simulink model "bh_motor_test_speed_and_thrust_RPS"  (R2016a)
settings: Solver=ode23s  StartTime=0.0  StopTime=10  FixedStep=0.001  RelTol=1e-5
undefined symbols (not defined in the file): P_mot, P_mot_alone, P_one_prop, sigbuilder_block
libraries: bh_6dof_LIBRARY x6
settings Model: Creator=bhorton  LastModifiedBy=bhorton
settings DataIOCC: SaveOutput=off  SignalLogging=off  DSMLogging=off  VisualizeSimOutput=off  SaveTime=off
settings DebuggingCC: AlgebraicLoopMsg=error  AllowSymbolicDim=off
settings ModelReferenceCC: PropagateSignalLabelsOutOfModel=off
settings GRTTargetCC: GeneratePreprocessorConditionals=Use local settings

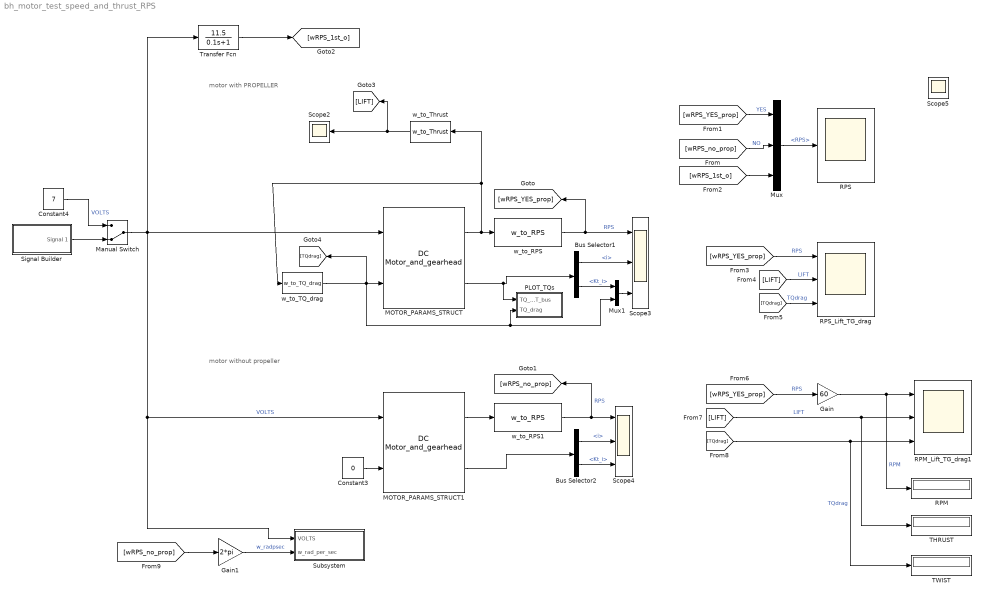
== system bh_motor_test_speed_and_thrust_RPS ==
  note: motor with PROPELLER
  note: motor without propeller
  Bus Selector1 : BusSelector  OutputSignals=Elec.i,TQ_mot.Kt_i
  Bus Selector2 : BusSelector  OutputSignals=Elec.i,TQ_mot.Kt_i
  Constant3 : Constant  Value=0
  Constant4 : Constant  Value=7
  Gain : Gain  Gain=60
  Gain1 : Gain  Gain=2*pi
  MOTOR_PARAMS_STRUCT : bh_6dof_LIBRARY/MODELS/DC Motor_and_gearhead  K=P_mot.Ka  B=P_mot.b  J=P_mot.I  R=P_mot.R  L=P_mot.L  Kb=P_mot.Ke  ID=P_mot.ID
  MOTOR_PARAMS_STRUCT1 : bh_6dof_LIBRARY/MODELS/DC Motor_and_gearhead  K=P_mot_alone.Ka  B=P_mot_alone.b  J=P_mot_alone.I  R=P_mot_alone.R  L=P_mot_alone.L  Kb=P_mot_alone.Ke  ID=P_mot.ID
  Manual Switch : ManualSwitch  CurrentSetting=0
  Mux : Mux  Inputs=3
  Mux1 : Mux  Inputs=2
  PLOT_TQs : Subsystem
  RPM : Display
  RPM_Lift_TG_drag1 : Scope  NumInputPorts=3
  RPS : Scope
  RPS_Lift_TG_drag : Scope  NumInputPorts=3
  Scope2 : Scope
  Scope3 : Scope  NumInputPorts=3
  Scope4 : Scope  NumInputPorts=3
  Signal Builder : Subsystem  Tag=STV Subsys  LoadFcn=sigbuilder_block('load');  StartFcn=sigbuilder_block('start');  StopFcn=sigbuilder_block('stop');  ClipboardFcn=sigbuilder_block('clipboard');  mask(Sigbuilder block){}
      mask help: Simulink:masks:SigbuilderBlock_MD
      mask init:
      | if ~strcmp(get_param(bdroot(gcbh),'SimulationStatus'),'stopped') tuvar = sigbuilder_block('maskInit'); end
      settings: CopyFcn=sigbuilder_block('copy');  DeleteFcn=sigbuilder_block('delete');  ModelCloseFcn=sigbuilder_block('modelClose');  PreSaveFcn=sigbuilder_block('preSave');  PauseFcn=sigbuilder_block('pause');  ContinueFcn=sigbuilder_block('continue');  NameChangeFcn=sigbuilder_block('namechange');  OpenFcn=sigbuilder_block('open',[536.25 210.75 551.25 360 ]);  CloseFcn=sigbuilder_block('close');
      mask Display: plot(0, 0, 100, 100,[2, 2, 32, 32, 2], [68, 8, 8, 68, 68],[32, 2], [38, 38], [32, 19, 2],[53, 60, 44], [32, 17, 17, 2],[16, 16, 31, 31]);txt = getActiveGroup(gcbh);text(2, 100, txt,'verticalAlignment', 'top');
  Subsystem : Subsystem
  THRUST : Display
  TWIST : Display
  Transfer Fcn : TransferFcn  Numerator=[0 11.5]  Denominator=[0.1 1]
  w_to_RPS : bh_6dof_LIBRARY/MODELS/w_to_RPS  SystemSampleTime=-1
  w_to_RPS1 : bh_6dof_LIBRARY/MODELS/w_to_RPS  SystemSampleTime=-1
  w_to_TQ_drag : bh_6dof_LIBRARY/MODELS/w_to_TQ_drag  k=P_one_prop.TWIST_per_w2
  w_to_Thrust : bh_6dof_LIBRARY/MODELS/w_to_Thrust  k=P_one_prop.LIFT_per_w2
  Scope5 : Scope
  wires:
  MOTOR_PARAMS_STRUCT/1 -> w_to_RPS/1, w_to_TQ_drag/1, w_to_Thrust/1
  w_to_RPS/1 -> [wRPS_YES_prop], Scope3/1  "RPS"
  MOTOR_PARAMS_STRUCT/2 -> PLOT_TQs/1(TQ_MOT_bus), Bus Selector1/1
  Bus Selector1/1 -> Scope3/2  "<i>"
  Bus Selector1/2 -> Mux1/1  "<Kt_i>"
  w_to_Thrust/1 -> [LIFT], Scope2/1
  MOTOR_PARAMS_STRUCT1/1 -> w_to_RPS1/1
  w_to_RPS1/1 -> [wRPS_no_prop], Scope4/1  "RPS"
  Manual Switch/1 -> Transfer Fcn/1, Subsystem/1(VOLTS), MOTOR_PARAMS_STRUCT1/1, MOTOR_PARAMS_STRUCT/1  "VOLTS"
  MOTOR_PARAMS_STRUCT1/2 -> Bus Selector2/1
  Bus Selector2/1 -> Scope4/2  "<i>"
  Bus Selector2/2 -> Scope4/3  "<Kt_i>"
  Constant3/1 -> MOTOR_PARAMS_STRUCT1/2
  [wRPS_no_prop] -> Mux/2  "NO"
  [wRPS_YES_prop] -> Mux/1  "YES"
  Mux/1 -> RPS/1  "<RPS>"
  Transfer Fcn/1 -> [wRPS_1st_o]
  [wRPS_1st_o] -> Mux/3
  Signal Builder/1(Signal 1) -> Manual Switch/2
  Constant4/1 -> Manual Switch/1  "VOLTS"
  [wRPS_YES_prop] -> RPS_Lift_TG_drag/1  "RPS"
  [LIFT] -> RPS_Lift_TG_drag/2  "LIFT"
  [TQdrag] -> RPS_Lift_TG_drag/3  "TQdrag"
  Mux1/1 -> Scope3/3
  w_to_TQ_drag/1 -> PLOT_TQs/2(TQ_drag), Mux1/2, [TQdrag], MOTOR_PARAMS_STRUCT/2
  [wRPS_YES_prop] -> Gain/1  "RPS"
  [LIFT] -> THRUST/1, RPM_Lift_TG_drag1/2  "LIFT"
  [TQdrag] -> TWIST/1, RPM_Lift_TG_drag1/3  "TQdrag"
  Gain/1 -> RPM/1, RPM_Lift_TG_drag1/1  "RPM"
  Gain1/1 -> Subsystem/2(w_rad_per_sec)  "w_radpsec"
  [wRPS_no_prop] -> Gain1/1

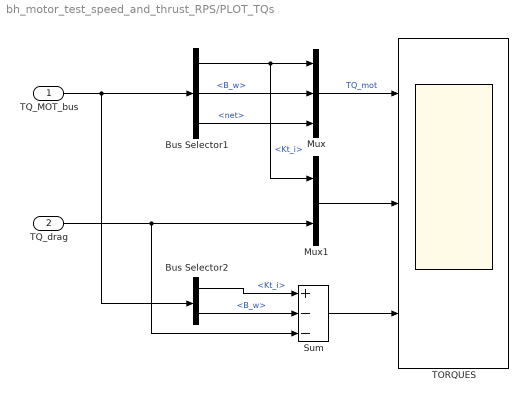
== system bh_motor_test_speed_and_thrust_RPS/PLOT_TQs ==
  TQ_MOT_bus : Inport
  TQ_drag : Inport  Port=2
  Bus Selector1 : BusSelector  OutputSignals=TQ_mot.Kt_i,TQ_mot.B_w,TQ_mot.net
  Bus Selector2 : BusSelector  OutputSignals=TQ_mot.Kt_i,TQ_mot.B_w
  Mux : Mux  Inputs=3
  Mux1 : Mux  Inputs=2
  Sum : Sum  Inputs=+|-|-
  TORQUES : Scope  NumInputPorts=3
  wires:
  TQ_MOT_bus/1 -> Bus Selector2/1, Bus Selector1/1
  Mux/1 -> TORQUES/1  "TQ_mot"
  Bus Selector1/1 -> Mux1/1, Mux/1  "<Kt_i>"
  Bus Selector1/3 -> Mux/3  "<net>"
  Bus Selector1/2 -> Mux/2  "<B_w>"
  Mux1/1 -> TORQUES/2
  Sum/1 -> TORQUES/3
  Bus Selector2/1 -> Sum/1  "<Kt_i>"
  Bus Selector2/2 -> Sum/2  "<B_w>"
  TQ_drag/1 -> Sum/3, Mux1/2

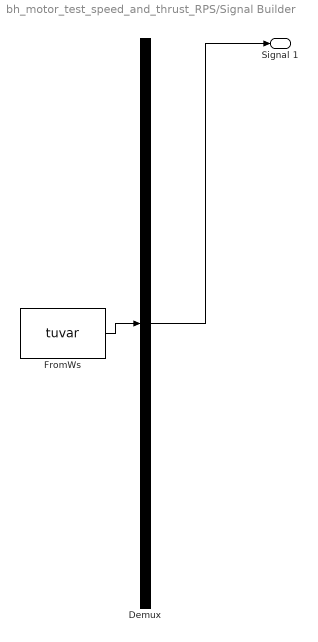
== system bh_motor_test_speed_and_thrust_RPS/Signal Builder ==
  Demux : Demux  Tag=STV Demux  Outputs=1
  FromWs : FromWorkspace  Tag=STV FromWs  VariableName=tuvar  SampleTime=0
      SigBuilderData=|
      | common.afterFinalStr = 'Extrapolate'
      | common.sampleTime = 0
      | dataSet(1).timeRange = [0 10]
      | dataSet(1).name = 'Group 1'
      | dataSet(2).timeRange = [0 10]
      | dataSet(2).name = 'Group 2'
      | sbobj.Groups(1).Name = 'Group 1'
      | sbobj.Groups(1).Signals.Name = 'Signal 1'
      | sbobj.Groups(1).Signals.XData = [0 1 1 2 2 3 3 4 4 5 5 6 6 7 7 8 8 9 9 10]
      | sbobj.Groups(1).Signals.YData = [0 0 1 1 2 2 3 3 4 4 5 5 6 6 7 7 8 8 9 9]
      | sbobj.Groups(2).Name = 'Group 2'
      | sbobj.Groups(2).Signals.Name = 'Signal 1'
      | sbobj.Groups(2).Signals.XData = [0 1 2 3 4 5 5 6 7 10]
      | sbobj.Groups(2).Signals.YData = [0 0 1 2 3 4 5 5 5 0]
  Signal 1 : Outport  Tag=STV Outport
  wires:
  Demux/1 -> Signal 1/1
  FromWs/1 -> Demux/1

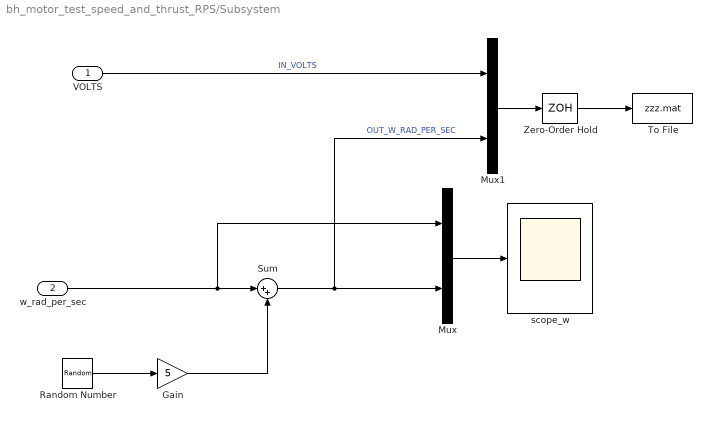
== system bh_motor_test_speed_and_thrust_RPS/Subsystem ==
  VOLTS : Inport
  w_rad_per_sec : Inport  Port=2
  Gain : Gain  Gain=5
  Mux : Mux  Inputs=2
  Mux1 : Mux  Inputs=2
  Random Number : RandomNumber  SampleTime=0.01
  Sum : Sum  Inputs=|++
  To File : ToFile  Filename=zzz.mat  MatrixName=MEAS_DATA_TS  SaveFormat=Timeseries
  Zero-Order Hold : ZeroOrderHold  SampleTime=0.01
  scope_w : Scope
  wires:
  Mux/1 -> scope_w/1
  w_rad_per_sec/1 -> Mux/1, Sum/1
  Random Number/1 -> Gain/1
  Gain/1 -> Sum/2
  Sum/1 -> Mux1/2, Mux/2  "OUT_W_RAD_PER_SEC"
  VOLTS/1 -> Mux1/1  "IN_VOLTS"
  Mux1/1 -> Zero-Order Hold/1
  Zero-Order Hold/1 -> To File/1
